simulink model "LATC_Test_Calc"  (R2021b)
settings: Solver=FixedStepDiscrete  StartTime=3849.7586  StopTime=3889.7825  FixedStep=0.01  RelTol=1e-3
values from neighbouring files (symbols this model uses):
  P_Global_CharSpd_ms : value not decoded    [PubParsGlobal.sldd]
  P_Global_SteeringAngleRatio : value not decoded    [PubParsGlobal.sldd]
  P_Global_WheelBase_m : value not decoded    [PubParsGlobal.sldd]
  P_LCS_CycleTime = 0.4 0.4 0.4 0.4 0.4 0.4 0.4 0.4 0.4 0.6 0.6 0.6 0.6 0.6 0.6 0.6 0.4 0.4 0.4 0.4 0.4 0.4 0.4 0.4 0.4 0.6 0.6 0.6 0.6 0.6 0.6 0.6 0.4 0.4 0.4 0.4 0.4 0.4 0.4 0.4 0.4 0.6 0.6 0.6 0.6 0.6 0.6 0.6 0.4 0.4 0.4 0.4 0.4 0.4 0.4 0.4 0.4 0.6 0.6 0.6 0.6 0.6 0.6 0.6 0.4 0.4 0.4 0.4 0.4 0.4 0.4 0.4 0.4 0.6 0.6 0.6 0.6 0.6 0.6 0.6 0.4 0.4 0.4 0.4 0.4 0.4 0.4 0.4 0.4 0.6 0.6 0.6 0.6 0.6 0.6 0.6 0.4 0.4 0.4 0.4    [LATC.sldd]
  P_LCS_ESS_AngleSlope_Limit = 2.9    [LATC.sldd]    (also in LCS_v05.sldd)
  P_LCS_LATC_CurOffsetVehicleSpdLimitValue_degs = 7.0    [LATC.sldd]
  P_LCS_LATC_ELKAngleSlope_ratio : value not decoded    [LATC.sldd]
  P_LCS_LATC_ELKMaxLatAcc_ms2 : value not decoded    [LATC.sldd]
  P_LCS_LATC_ESSAngleSlope_ratio : value not decoded    [LATC.sldd]
  P_LCS_LATC_ESSMaxLatAcc_ms2 : value not decoded    [LATC.sldd]
  P_LCS_LATC_LCAngleSlope_ratio : value not decoded    [LATC.sldd]
  P_LCS_LATC_LCCancleMaxLatAcc_ms2 : value not decoded    [LATC.sldd]
  P_LCS_LATC_LCEcoAngleSlope_ratio : value not decoded    [LATC.sldd]
  P_LCS_LATC_LCEcoMaxLatAcc_ms2 : value not decoded    [LATC.sldd]
  P_LCS_LATC_LCKAngleSlope_ratio : value not decoded    [LATC.sldd]
  P_LCS_LATC_LCKIEAngleSlope_ratio : value not decoded    [LATC.sldd]
  P_LCS_LATC_LCKIEMaxLatAcc_ms2 : value not decoded    [LATC.sldd]
  P_LCS_LATC_LCKMaxLatAcc_ms2 : value not decoded    [LATC.sldd]
  P_LCS_LATC_LCNormalAngleSlope_ratio : value not decoded    [LATC.sldd]
  P_LCS_LATC_LCNormalMaxLatAcc_ms2 : value not decoded    [LATC.sldd]
  P_LCS_LATC_LCSportAngleSlope_ratio : value not decoded    [LATC.sldd]
  P_LCS_LATC_LCSportMaxLatAcc_ms2 : value not decoded    [LATC.sldd]
  P_LCS_LATC_LKAAngleSlope_ratio : value not decoded    [LATC.sldd]
  P_LCS_LATC_LKAMaxLatAcc_ms2 : value not decoded    [LATC.sldd]
  P_LCS_LATC_MatrixQ1_st = 0.8 0.8 1.2 1.4 1.4 1.4 2.0 2.2 2.2 2.2 2.2 2.2 2.2 2.2 2.2 2.2 0.8 0.8 1.2 1.4 1.4 1.4 2.0 2.2 2.2 2.2 2.2 2.2 2.2 2.2 2.2 2.2 0.8 0.8 1.2 1.4 1.4 1.4 2.0 2.2 2.2 2.2 2.2 2.2 2.2 2.2 2.2 2.2 0.8 0.8 1.2 1.4 1.4 1.4 2.0 2.2 2.2 2.2 2.2 2.2 2.2 2.2 2.2 2.2 0.8 0.8 1.2 1.4 1.4 1.4 2.0 2.2 2.2 2.2 2.2 2.2 2.2 2.2 2.2 2.2 0.8 0.8 1.2 1.4 1.4 1.4 2.0 2.2 2.2 2.2 2.2 2.2 2.2 2.2 2.2 2.2 0.8 0.8 1.2 1.4    [LATC.sldd]
  P_LCS_LATC_MatrixQ3_st = 20.0 20.0 20.0 20.0 20.0 15.0 15.0 15.0 15.0 15.0 15.0 15.0 15.0 13.0 13.0 13.0 20.0 20.0 20.0 20.0 20.0 15.0 15.0 15.0 15.0 15.0 15.0 15.0 15.0 13.0 13.0 13.0 20.0 20.0 20.0 20.0 20.0 15.0 15.0 15.0 15.0 15.0 15.0 15.0 15.0 13.0 13.0 13.0 20.0 20.0 20.0 20.0 20.0 15.0 15.0 15.0 15.0 15.0 15.0 15.0 15.0 13.0 13.0 13.0 20.0 20.0 20.0 20.0 20.0 15.0 15.0 15.0 15.0 15.0 15.0 15.0 15.0 13.0 13.0 13.0    [LATC.sldd]
  P_LCS_LATC_MatrixR_st = 10.0 10.0 10.0 10.0 10.0 10.0 10.0 15.0 15.0 15.0 15.0 15.0 15.0 15.0 15.0 15.0 10.0 10.0 10.0 10.0 10.0 10.0 10.0 15.0 15.0 15.0 15.0 15.0 15.0 15.0 15.0 15.0 10.0 10.0 10.0 10.0 10.0 10.0 10.0 15.0 15.0 15.0 15.0 15.0 15.0 15.0 15.0 15.0 10.0 10.0 10.0 10.0 10.0 10.0 10.0 15.0 15.0 15.0 15.0 15.0 15.0 15.0 15.0 15.0 10.0 10.0 10.0 10.0 10.0 10.0 10.0 15.0 15.0 15.0 15.0 15.0 15.0 15.0 15.0 15.0    [LATC.sldd]
  P_LCS_LATC_StateActivAngleSlopeLimit_ratio : value not decoded    [LATC.sldd]
  P_LCS_LATC_StateActiveFlg_TabX_st : value not decoded    [LATC.sldd]
  P_LCS_LATC_StateActiveHoldTime_TabY_st : value not decoded    [LATC.sldd]
  P_LCS_LATC_StateHoldTime_st = 250.0    [LATC.sldd]
  P_LCS_LATC_TarAngleFliterWindowSize = 5.0    [LATC.sldd]
  P_LCS_LineVaildSW = 0.0    [LATC.sldd]
  P_LCS_Lookahead_Distance : value not decoded    [LATC.sldd]
  P_LCS_VehicleSpd_TabX_Kph : value not decoded    [LATC.sldd]
libraries: simulink x4
(part 2 of 4)

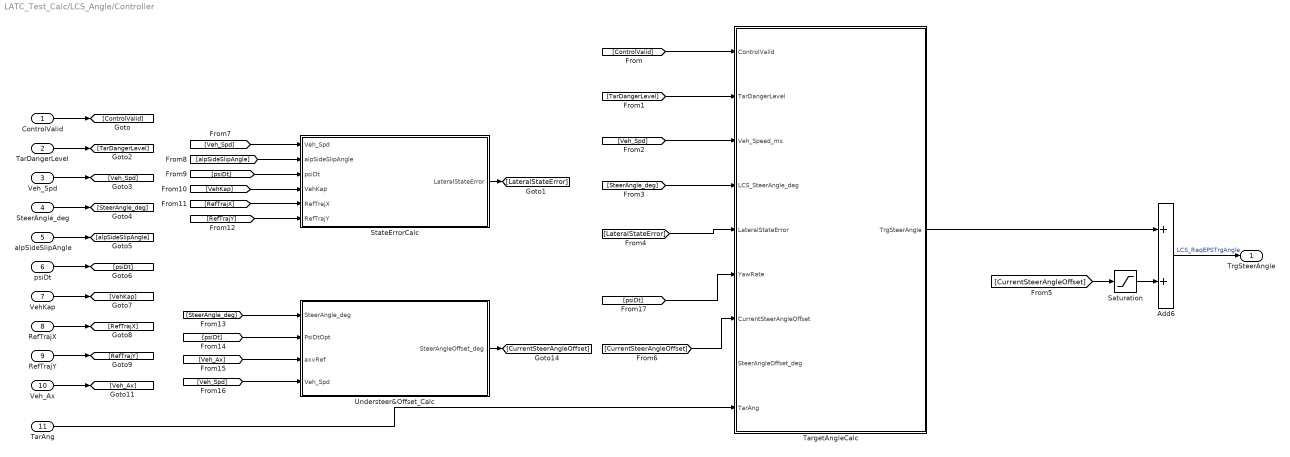
== system LATC_Test_Calc/LCS_Angle/Controller ==
  ControlValid : Inport
  TarDangerLevel : Inport  Port=2
  Veh_Spd : Inport  Port=3
  SteerAngle_deg : Inport  Port=4
  alpSideSlipAngle : Inport  Port=5
  psiDt : Inport  Port=6
  VehKap : Inport  Port=7
  RefTrajX : Inport  Port=8
  RefTrajY : Inport  Port=9
  Veh_Ax : Inport  Port=10
  TarAng : Inport  Port=11
  Add6 : Sum  AccumDataTypeStr=single
  Saturation : Saturate  UpperLimit=10  LowerLimit=-10
  StateErrorCalc : Subsystem
  TargetAngleCalc : Subsystem
  Understeer&Offset_Calc : Subsystem
  TrgSteerAngle : Outport
  wires:
  Understeer&Offset_Calc/1(SteerAngleOffset_deg) -> [CurrentSteerAngleOffset]
  StateErrorCalc/1(LateralStateError) -> [LateralStateError]
  ControlValid/1 -> [ControlValid]
  TarDangerLevel/1 -> [TarDangerLevel]
  Veh_Spd/1 -> [Veh_Spd]
  SteerAngle_deg/1 -> [SteerAngle_deg]
  alpSideSlipAngle/1 -> [alpSideSlipAngle]
  psiDt/1 -> [psiDt]
  VehKap/1 -> [VehKap]
  RefTrajX/1 -> [RefTrajX]
  RefTrajY/1 -> [RefTrajY]
  [ControlValid] -> TargetAngleCalc/1(ControlValid)
  [TarDangerLevel] -> TargetAngleCalc/2(TarDangerLevel)
  [Veh_Spd] -> TargetAngleCalc/3(Veh_Speed_ms)
  [SteerAngle_deg] -> TargetAngleCalc/4(LCS_SteerAngle_deg)
  [LateralStateError] -> TargetAngleCalc/5(LateralStateError)
  [psiDt] -> TargetAngleCalc/6(YawRate)
  [CurrentSteerAngleOffset] -> TargetAngleCalc/7(CurrentSteerAngleOffset)
  [Veh_Spd] -> StateErrorCalc/1(Veh_Spd)
  [alpSideSlipAngle] -> StateErrorCalc/2(alpSideSlipAngle)
  [psiDt] -> StateErrorCalc/3(psiDt)
  [VehKap] -> StateErrorCalc/4(VehKap)
  [RefTrajX] -> StateErrorCalc/5(RefTrajX)
  [RefTrajY] -> StateErrorCalc/6(RefTrajY)
  [SteerAngle_deg] -> Understeer&Offset_Calc/1(SteerAngle_deg)
  [psiDt] -> Understeer&Offset_Calc/2(PsiDtOpt)
  Veh_Ax/1 -> [Veh_Ax]
  [Veh_Ax] -> Understeer&Offset_Calc/3(axvRef)
  [Veh_Spd] -> Understeer&Offset_Calc/4(Veh_Spd)
  [CurrentSteerAngleOffset] -> Saturation/1
  Saturation/1 -> Add6/2
  TargetAngleCalc/1(TrgSteerAngle) -> Add6/1
  Add6/1 -> TrgSteerAngle/1  "LCS_ReqEPSTrgAngle"
  TarAng/1 -> TargetAngleCalc/9(TarAng)

== system LATC_Test_Calc/LCS_Angle/LaneWidthFac ==
  LaneWidth : Inport
  Constant4 : Constant  Value=3.6  OutDataTypeStr=single
  Constant6 : Constant  Value=3  OutDataTypeStr=single
  Constant7 : Constant  Value=4  OutDataTypeStr=single
  Divide1 : Product  Inputs=*/
  MinMax : MinMax  Function=max  Inputs=2
  MinMax1 : MinMax  Inputs=2
  LaneWidthFac : Outport
  wires:
  LaneWidth/1 -> MinMax/1
  Constant7/1 -> MinMax1/2
  MinMax/1 -> MinMax1/1
  Constant6/1 -> MinMax/2
  Constant4/1 -> Divide1/2
  MinMax1/1 -> Divide1/1
  Divide1/1 -> LaneWidthFac/1

== system LATC_Test_Calc/LCS_Angle/Subsystem ==
  canSteerWheelSpd : Inport
  canSteerWheelSpdSign : Inport  Port=2
  Bias2 : Bias  Bias=-0.5
  Gain2 : Gain  Gain=-2
  Product4 : Product
  LCS_IN_SteerAngleSpd_degs : Outport
  wires:
  Gain2/1 -> Product4/2
  Product4/1 -> LCS_IN_SteerAngleSpd_degs/1
  canSteerWheelSpdSign/1 -> Bias2/1
  Bias2/1 -> Gain2/1
  canSteerWheelSpd/1 -> Product4/1

== system LATC_Test_Calc/LCS_Angle/Subsystem1 ==
  Speed_ms : Inport
  Constant8 : Constant  Value=1.3  OutDataTypeStr=single
  Gain3 : Gain  Gain=3.6
  Gain4 : Gain  Gain=1.03
  Sum : Sum
  LCS_DisplaySpd_kph : Outport
  wires:
  Constant8/1 -> Sum/2
  Speed_ms/1 -> Gain3/1
  Gain3/1 -> Gain4/1
  Sum/1 -> LCS_DisplaySpd_kph/1
  Gain4/1 -> Sum/1

== system LATC_Test_Calc/LCS_Angle/Subsystem3 ==
  canSteerWheelAngle : Inport
  canSteerWheelAngleSign : Inport  Port=2
  Bias1 : Bias  Bias=-0.5
  Gain5 : Gain  Gain=-2
  Product5 : Product
  LCS_IN_CurSteerAngle_deg : Outport
  wires:
  Bias1/1 -> Gain5/1
  canSteerWheelAngle/1 -> Product5/1
  Gain5/1 -> Product5/2
  canSteerWheelAngleSign/1 -> Bias1/1
  Product5/1 -> LCS_IN_CurSteerAngle_deg/1  "LCS_IN_CurSteerAngle_deg"

== system LATC_Test_Calc/LCS_Angle/Subsystem5 ==
  raw : Inport
  Slope : Inport  Port=2
  Add : Sum
  Add1 : Sum  Inputs=+-
  Max : MinMax  Inputs=2
  Min : MinMax  Function=max  Inputs=2
  Unit Delay : UnitDelay  InitialCondition=single(0)  SampleTime=-1  HasFrameUpgradeWarning=on
  out : Outport
  wires:
  raw/1 -> Max/2
  Add1/1 -> Min/2
  Add/1 -> Max/1
  Max/1 -> Min/1
  Min/1 -> Unit Delay/1, out/1
  Unit Delay/1 -> Add/1, Add1/1
  Slope/1 -> Add/2, Add1/2

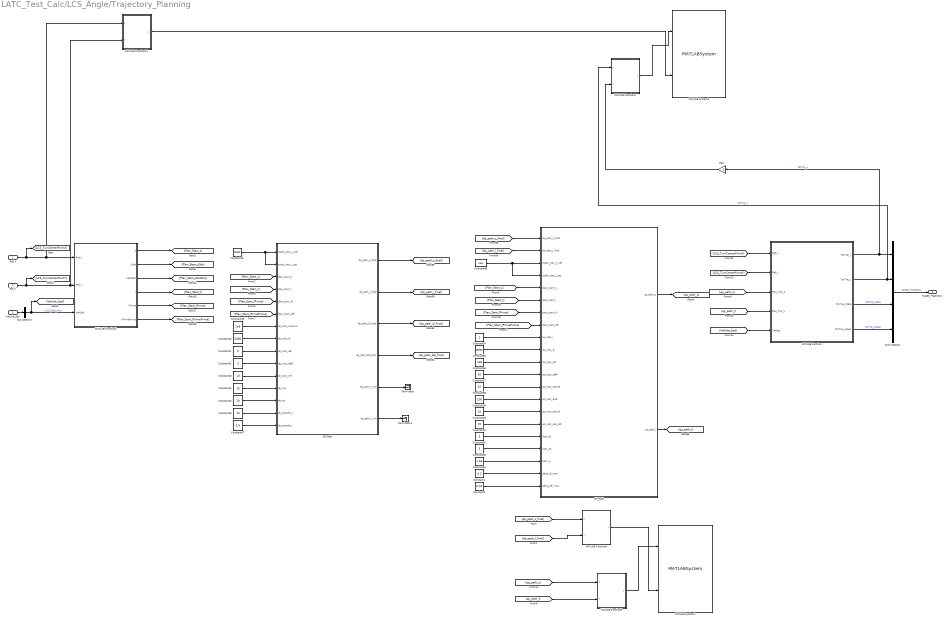
== system LATC_Test_Calc/LCS_Angle/Trajectory_Planning ==
  Ref_X : Inport
  Ref_Y : Inport  Port=2
  Vehicle_Spd : Inport  Port=3
  Bus Creator1 : BusCreator  Inputs=4
  Bus Selector : BusSelector  OutputSignals=LCS_Spd_ms
  Constant1 : Constant  Value=0.2  OutDataTypeStr=single
  Constant2 : Constant  Value=0.01  OutDataTypeStr=single
  Constant39 : Constant  Value=1e9  OutDataTypeStr=single
  Constant40 : Constant  Value=2000  OutDataTypeStr=single
  Constant41 : Constant  Value=2  OutDataTypeStr=single
  Constant42 : Constant  Value=3  OutDataTypeStr=single
  Constant43 : Constant  Value=10  OutDataTypeStr=single
  Constant{44,58,60..61} (4 alike) : Constant  Value=15  OutDataTypeStr=single
  Constant45 : Constant  Value=10  OutDataTypeStr=single
  Constant46 : Constant  Value=12  OutDataTypeStr=single
  Constant47 : Constant  Value=0.5  OutDataTypeStr=single
  Constant49 : Constant  Value=NaN  OutDataTypeStr=single
  Constant54 : Constant  OutDataTypeStr=single
  Constant55 : Constant  Value=25000  OutDataTypeStr=single
  Constant56 : Constant  Value=100  OutDataTypeStr=single
  Constant57 : Constant  Value=20  OutDataTypeStr=single
  Constant59 : Constant  Value=100  OutDataTypeStr=single
  Constant62 : Constant  Value=3  OutDataTypeStr=single
  Constant63 : Constant  Value=3  OutDataTypeStr=single
  Constant64 : Constant  Value=1.63  OutDataTypeStr=single
  Constant68 : Constant  Value=nan  OutDataTypeStr=single
  DP_Path : Subsystem
  Gain : Gain  Gain=-1
  MATLAB Function : MATLAB Function  TreatAsAtomicUnit=on
  MATLAB Function1 : MATLAB Function  TreatAsAtomicUnit=on
  MATLAB Function14 : MATLAB Function  TreatAsAtomicUnit=on
  MATLAB Function2 : MATLAB Function  TreatAsAtomicUnit=on
  MATLAB Function3 : MATLAB Function  TreatAsAtomicUnit=on
  MATLAB Function4 : MATLAB Function  TreatAsAtomicUnit=on
  MATLAB System1 : MATLABSystem  System=BirdsEyeView17a  XLim=[ 0, 120 ]  YLim=[ -30, 30 ]  HasActors=off  ActorsColor=off  HasVision=on  HasRadar=on  HasRoads=off  HasLaneMarkings=off  Camera_Fov=52  Camera_Range=100  Camera_Yaw=0  Camera_Pos=[ 0, 0 ]  Radar_Fov=52  Radar_Range=100  Radar_Yaw=0  Radar_Pos=[ 0, 0 ]  MarkerSize=4  LabelFontSize=4  LabelOffset=[ 1.5, 1.5 ]  aspectratio=off
      mask Type: BirdsEyeView17a
      mask Display:
      | disp(['Bird''s-Eye' char(10) 'View']);
      | port_label('input',1,'Vision');
      | port_label('input',2,'Radar');
  MATLAB System3 : MATLABSystem  System=BirdsEyeView17a  XLim=[ 0, 120 ]  YLim=[ -30, 30 ]  HasActors=off  ActorsColor=off  HasVision=on  HasRadar=on  HasRoads=off  HasLaneMarkings=off  Camera_Fov=52  Camera_Range=100  Camera_Yaw=0  Camera_Pos=[ 0, 0 ]  Radar_Fov=52  Radar_Range=100  Radar_Yaw=0  Radar_Pos=[ 0, 0 ]  MarkerSize=4  LabelFontSize=4  LabelOffset=[ 1.5, 1.5 ]  aspectratio=off
      mask Type: BirdsEyeView17a
      mask Display:
      | disp(['Bird''s-Eye' char(10) 'View']);
      | port_label('input',1,'Vision');
      | port_label('input',2,'Radar');
  QP_Path : Subsystem
  Terminator : Terminator
  Terminator1 : Terminator
  Target_Trajectory : Outport
  wires:
  Constant55/1 -> QP_Path/10(qp_cost_dl)
  MATLAB Function2/6(lPrimePrime) -> [Plan_Start_lPrimePrime]
  MATLAB Function2/1(s) -> [Plan_Start_s]
  Constant41/1 -> DP_Path/9(dp_cost_ddl)
  Constant56/1 -> QP_Path/11(qp_cost_ddl)
  QP_Path/2(qp_path_l) -> [qp_path_l]
  [Plan_Start_lPrime] -> DP_Path/5(plan_start_dl)
  Constant62/1 -> QP_Path/17(host_d1)
  Constant61/1 -> QP_Path/16(qp_cost_end_ddl)
  [Plan_Start_lPrimePrime] -> DP_Path/6(plan_start_ddl)
  Constant54/1 -> QP_Path/9(qp_cost_l)
  Constant42/1 -> DP_Path/10(dp_cost_dddl)
  Vehicle_Spd/1 -> Bus Selector/1
  [Plan_Start_lPrimePrime] -> QP_Path/8(plan_start_ddl)
  Constant59/1 -> QP_Path/14(qp_cost_endl)
  Constant68/1 -> QP_Path/4(static_obs_l_set), QP_Path/3(static_obs_s_set)
  Constant44/1 -> DP_Path/12(dp_row)
  [Plan_Start_l] -> DP_Path/4(plan_start_l)
  MATLAB Function2/5(lPrime) -> [Plan_Start_lPrime]
  [Plan_Start_s] -> DP_Path/3(plan_start_s)
  DP_Path/1(dp_path_s_final) -> [dp_path_s_final]
  [dp_path_s_final] -> QP_Path/1(dp_path_s_final)
  Constant64/1 -> QP_Path/19(host_w)
  MATLAB Function2/3(sDotDot) -> [Plan_Start_sDotDot]
  Constant46/1 -> DP_Path/14(dp_sample_s)
  [Vehicle_Spd] -> MATLAB Function/5(VehSpd)
  Constant63/1 -> QP_Path/18(host_d2)
  DP_Path/3(dp_path_dl_final) -> [dp_path_dl_final]
  DP_Path/2(dp_path_l_final) -> [dp_path_l_final]
  Constant40/1 -> DP_Path/8(dp_cost_dl)
  Constant57/1 -> QP_Path/12(qp_cost_dddl)
  Constant47/1 -> DP_Path/15(dp_sample_l)
  MATLAB Function2/4(l) -> [Plan_Start_l]
  MATLAB Function2/2(sDot) -> [Plan_Start_sDot]
  Constant39/1 -> DP_Path/7(dp_cost_collision)
  Constant43/1 -> DP_Path/11(dp_cost_ref)
  [Plan_Start_lPrime] -> QP_Path/7(plan_start_dl)
  MATLAB Function/1(TarTraj_x) -> Gain/1, Bus Creator1/1  "TarTraj_x"
  DP_Path/4(dp_path_ddl_final) -> [dp_path_ddl_final]
  Constant60/1 -> QP_Path/15(qp_cost_end_dl)
  [LCS_TurnCenterPointY] -> MATLAB Function/2(Ref_Y)
  Bus Selector/1 -> [Vehicle_Spd], MATLAB Function2/3(VehSpd)  "<LCS_Spd_ms>"
  [Plan_Start_l] -> QP_Path/6(plan_start_l)
  [qp_path_s] -> MATLAB Function/3(Plan_Traj_S)
  DP_Path/6(dp_path_l_init) -> Terminator1/1
  Constant49/1 -> DP_Path/2(static_obs_l_set), DP_Path/1(static_obs_s_set)
  Constant58/1 -> QP_Path/13(qp_cost_centre)
  [dp_path_l_final] -> QP_Path/2(dp_path_l_final)
  DP_Path/5(dp_path_s_init) -> Terminator/1
  Constant45/1 -> DP_Path/13(dp_col)
  [qp_path_l] -> MATLAB Function/4(Plan_Traj_L)
  Bus Creator1/1 -> Target_Trajectory/1  "Target_Trajectory"
  [LCS_TurnCenterPointX] -> MATLAB Function/1(Ref_X)
  MATLAB Function/4(TarTraj_kappa) -> Bus Creator1/4  "TarTraj_kappa"
  MATLAB Function/2(TarTraj_y) -> MATLAB Function1/1(X), Bus Creator1/2  "TarTraj_y"
  MATLAB Function/3(TarTraj_theta) -> Bus Creator1/3  "TarTraj_theta"
  Ref_X/1 -> [LCS_TurnCenterPointX], MATLAB Function14/1(X), MATLAB Function2/1(Ref_X)
  MATLAB Function1/1(y) -> MATLAB System3/1
  Ref_Y/1 -> [LCS_TurnCenterPointY], MATLAB Function14/2(Y), MATLAB Function2/2(Ref_Y)
  MATLAB Function14/1(y) -> MATLAB System3/2
  Gain/1 -> MATLAB Function1/2(Y)
  [dp_path_l_final] -> MATLAB Function4/2(Y)
  MATLAB Function3/1(y) -> MATLAB System1/1
  [dp_path_s_final] -> MATLAB Function4/1(X)
  MATLAB Function4/1(y) -> MATLAB System1/2
  Constant1/1 -> QP_Path/20(delta_dl_max)
  Constant2/1 -> QP_Path/21(delta_ddl_max)
  QP_Path/1(qp_path_s) -> [qp_path_s]
  [Plan_Start_s] -> QP_Path/5(plan_start_s)
  [qp_path_s] -> MATLAB Function3/1(X)
  [qp_path_l] -> MATLAB Function3/2(Y)

== system LATC_Test_Calc/LCS_Angle/Trajectory_Points ==
  A0 : Inport
  A1 : Inport  Port=2
  A2 : Inport  Port=3
  A3 : Inport  Port=4
  LineVaild : Inport  Port=5
  MATLAB Function1 : MATLAB Function  TreatAsAtomicUnit=on
  RoadCreate1 : Subsystem
  LCS_TurnCenterPointX : Outport
  LCS_TurnCenterPointY : Outport  Port=2
  Control_Valid : Outport  Port=3
  wires:
  A1/1 -> RoadCreate1/2(A1)
  MATLAB Function1/2(CenterLinePoint2_Y) -> LCS_TurnCenterPointY/1  "LCS_TurnCenterPointY"
  A0/1 -> RoadCreate1/1(A0)
  MATLAB Function1/1(CenterLinePoint2_X) -> LCS_TurnCenterPointX/1  "LCS_TurnCenterPointX"
  A2/1 -> RoadCreate1/3(A2)
  LineVaild/1 -> RoadCreate1/5(LineVaild)
  RoadCreate1/3(Control_Valid) -> Control_Valid/1
  A3/1 -> RoadCreate1/4(A3)
  RoadCreate1/1(CenterLinePointX) -> MATLAB Function1/1(CenterLinePointX)
  RoadCreate1/2(CenterLinePointY) -> MATLAB Function1/2(CenterLinePointY)

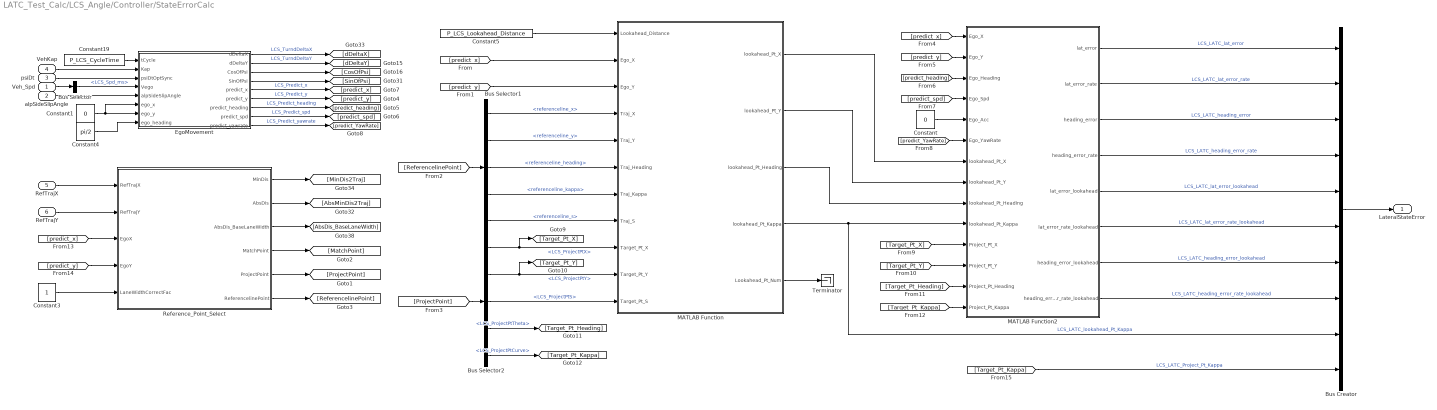
== system LATC_Test_Calc/LCS_Angle/Controller/StateErrorCalc ==
  Veh_Spd : Inport
  alpSideSlipAngle : Inport  Port=2
  psiDt : Inport  Port=3
  VehKap : Inport  Port=4
  RefTrajX : Inport  Port=5
  RefTrajY : Inport  Port=6
  Bus Creator : BusCreator  Inputs=10
  Bus Selector : BusSelector  OutputSignals=LCS_Spd_ms
  Bus Selector1 : BusSelector  OutputSignals=referenceline_x,referenceline_y,referenceline_heading,referenceline_kappa,referenceline_s
  Bus Selector2 : BusSelector  OutputSignals=LCS_ProjectPtX,LCS_ProjectPtY,LCS_ProjectPtS,LCS_ProjectPtTheta,LCS_ProjectPtCurve
  Constant : Constant  Value=0  OutDataTypeStr=single
  Constant1 : Constant  Value=0  OutDataTypeStr=single
  Constant19 : Constant  Value=P_LCS_CycleTime  OutDataTypeStr=single
  Constant3 : Constant  OutDataTypeStr=single
  Constant4 : Constant  Value=pi/2  OutDataTypeStr=single
  Constant5 : Constant  Value=P_LCS_Lookahead_Distance  OutDataTypeStr=single
  EgoMovement : MATLAB Function  TreatAsAtomicUnit=on
  MATLAB Function : MATLAB Function  TreatAsAtomicUnit=on
  MATLAB Function2 : MATLAB Function  TreatAsAtomicUnit=on
  Reference_Point_Select : Subsystem
  Terminator : Terminator
  LateralStateError : Outport
  wires:
  Constant19/1 -> EgoMovement/1(tCycle)
  Bus Selector/1 -> EgoMovement/4(Vego)  "<LCS_Spd_ms>"
  EgoMovement/1(dDeltaX) -> [dDeltaX]  "LCS_TurndDeltaX"
  EgoMovement/4(SinOfPsi) -> [SinOfPsi]
  VehKap/1 -> EgoMovement/2(Kap)
  EgoMovement/3(CosOfPsi) -> [CosOfPsi]
  Veh_Spd/1 -> Bus Selector/1
  alpSideSlipAngle/1 -> EgoMovement/5(alpSideSlipAngle)
  psiDt/1 -> EgoMovement/3(psiDtOptSync)
  EgoMovement/2(dDeltaY) -> [dDeltaY]  "LCS_TurndDeltaY"
  Reference_Point_Select/3(AbsDis_BaseLaneWidth) -> [AbsDis_BaseLaneWidth]
  Reference_Point_Select/2(AbsDis) -> [AbsMinDis2Traj]
  Reference_Point_Select/1(MinDis) -> [MinDis2Traj]
  RefTrajX/1 -> Reference_Point_Select/1(RefTrajX)
  Constant3/1 -> Reference_Point_Select/5(LaneWidthCorrectFac)
  RefTrajY/1 -> Reference_Point_Select/2(RefTrajY)
  Reference_Point_Select/4(MatchPoint) -> [MatchPoint]
  Reference_Point_Select/5(ProjectPoint) -> [ProjectPoint]
  Reference_Point_Select/6(ReferencelinePoint) -> [ReferencelinePoint]
  EgoMovement/5(predict_x) -> [predict_x]  "LCS_Predict_x"
  EgoMovement/6(predict_y) -> [predict_y]  "LCS_Predict_y"
  EgoMovement/7(predict_heading) -> [predict_heading]  "LCS_Predict_heading"
  EgoMovement/8(predict_spd) -> [predict_spd]  "LCS_Predict_spd"
  EgoMovement/9(predict_yawrate) -> [predict_YawRate]  "LCS_Predict_yawrate"
  [predict_x] -> MATLAB Function/2(Ego_X)
  [predict_y] -> MATLAB Function/3(Ego_Y)
  [ReferencelinePoint] -> Bus Selector1/1
  Bus Selector1/1 -> MATLAB Function/4(Traj_X)  "<referenceline_x>"
  Bus Selector1/2 -> MATLAB Function/5(Traj_Y)  "<referenceline_y>"
  Bus Selector1/3 -> MATLAB Function/6(Traj_Heading)  "<referenceline_heading>"
  Bus Selector1/4 -> MATLAB Function/7(Traj_Kappa)  "<referenceline_kappa>"
  Bus Selector1/5 -> MATLAB Function/8(Traj_S)  "<referenceline_s>"
  [ProjectPoint] -> Bus Selector2/1
  Bus Selector2/2 -> [Target_Pt_Y], MATLAB Function/10(Target_Pt_Y)  "<LCS_ProjectPtY>"
  Bus Selector2/1 -> [Target_Pt_X], MATLAB Function/9(Target_Pt_X)  "<LCS_ProjectPtX>"
  Bus Selector2/3 -> MATLAB Function/11(Target_Pt_S)  "<LCS_ProjectPtS>"
  [predict_x] -> MATLAB Function2/1(Ego_X)
  [predict_y] -> MATLAB Function2/2(Ego_Y)
  [predict_heading] -> MATLAB Function2/3(Ego_Heading)
  [predict_spd] -> MATLAB Function2/4(Ego_Spd)
  [predict_YawRate] -> MATLAB Function2/6(Ego_YawRate)
  Constant/1 -> MATLAB Function2/5(Ego_Acc)
  Bus Selector2/4 -> [Target_Pt_Heading]  "<LCS_ProjectPtTheta>"
  Bus Selector2/5 -> [Target_Pt_Kappa]  "<LCS_ProjectPtCurve>"
  [Target_Pt_X] -> MATLAB Function2/11(Project_Pt_X)
  [Target_Pt_Y] -> MATLAB Function2/12(Project_Pt_Y)
  [Target_Pt_Heading] -> MATLAB Function2/13(Project_Pt_Heading)
  [Target_Pt_Kappa] -> MATLAB Function2/14(Project_Pt_Kappa)
  Constant1/1 -> EgoMovement/7(ego_y), EgoMovement/6(ego_x)
  MATLAB Function2/4(heading_error_rate) -> Bus Creator/4  "LCS_LATC_heading_error_rate"
  MATLAB Function2/2(lat_error_rate) -> Bus Creator/2  "LCS_LATC_lat_error_rate"
  MATLAB Function2/3(heading_error) -> Bus Creator/3  "LCS_LATC_heading_error"
  MATLAB Function2/1(lat_error) -> Bus Creator/1  "LCS_LATC_lat_error"
  Bus Creator/1 -> LateralStateError/1
  Constant4/1 -> EgoMovement/8(ego_heading)
  MATLAB Function/4(lookahead_Pt_Kappa) -> Bus Creator/9, MATLAB Function2/10(lookahead_Pt_Kappa)  "LCS_LATC_lookahead_Pt_Kappa"
  Constant5/1 -> MATLAB Function/1(Lookahead_Distance)
  [predict_x] -> Reference_Point_Select/3(EgoX)
  [predict_y] -> Reference_Point_Select/4(EgoY)
  MATLAB Function/5(Lookahead_Pt_Num) -> Terminator/1
  MATLAB Function/2(lookahead_Pt_Y) -> MATLAB Function2/8(lookahead_Pt_Y)
  MATLAB Function/1(lookahead_Pt_X) -> MATLAB Function2/7(lookahead_Pt_X)
  MATLAB Function/3(lookahead_Pt_Heading) -> MATLAB Function2/9(lookahead_Pt_Heading)
  MATLAB Function2/5(lat_error_lookahead) -> Bus Creator/5  "LCS_LATC_lat_error_lookahead"
  MATLAB Function2/6(lat_error_rate_lookahead) -> Bus Creator/6  "LCS_LATC_lat_error_rate_lookahead"
  MATLAB Function2/7(heading_error_lookahead) -> Bus Creator/7  "LCS_LATC_heading_error_lookahead"
  MATLAB Function2/8(heading_error_rate_lookahead) -> Bus Creator/8  "LCS_LATC_heading_error_rate_lookahead"
  [Target_Pt_Kappa] -> Bus Creator/10  "LCS_LATC_Project_Pt_Kappa"

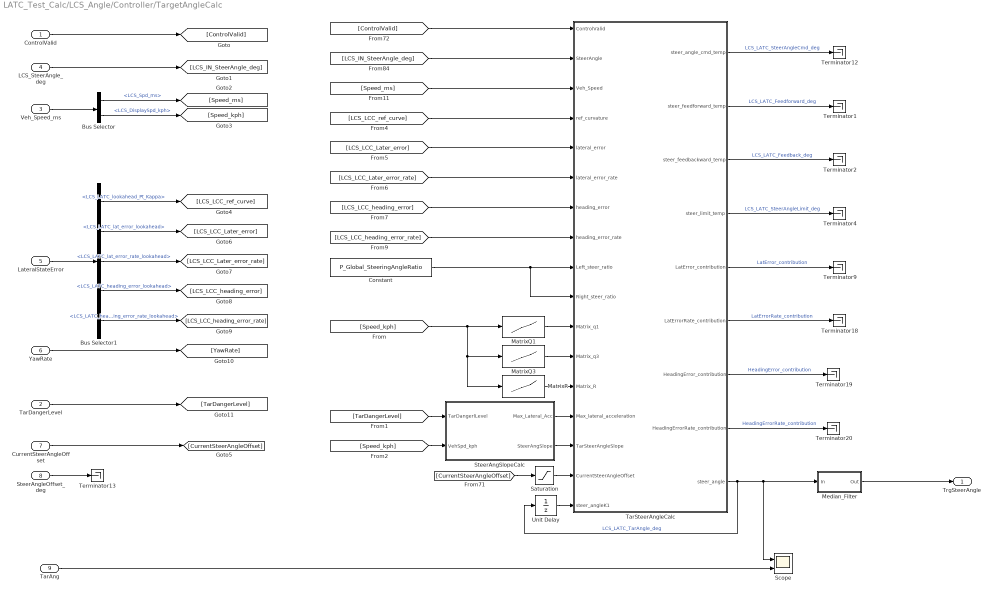
== system LATC_Test_Calc/LCS_Angle/Controller/TargetAngleCalc ==
  ControlValid : Inport
  TarDangerLevel : Inport  Port=2
  Veh_Speed_ms : Inport  Port=3
  LCS_SteerAngle_deg : Inport  Port=4
  LateralStateError : Inport  Port=5
  YawRate : Inport  Port=6
  CurrentSteerAngleOffset : Inport  Port=7
  SteerAngleOffset_deg : Inport  Port=8
  TarAng : Inport  Port=9
  Bus Selector : BusSelector  OutputSignals=LCS_Spd_ms,LCS_DisplaySpd_kph
  Bus Selector1 : BusSelector  OutputSignals=LCS_LATC_lookahead_Pt_Kappa,LCS_LATC_lat_error_lookahead,LCS_LATC_lat_error_rate_lookahead,LCS_LATC_heading_error_lookahead,LCS_LATC_heading_error_rate_lookahead
  Constant : Constant  Value=P_Global_SteeringAngleRatio  OutDataTypeStr=single
  MatrixQ1 : Lookup_n-D  NumberOfTableDimensions=1  BreakpointsForDimension1=P_LCS_VehicleSpd_TabX_Kph  Table=P_LCS_LATC_MatrixQ1_st  ExtrapMethod=Clip  UseLastTableValue=on  InternalRulePriority=Speed  RndMeth=Simplest  InputSameDT=on
  MatrixQ3 : Lookup_n-D  NumberOfTableDimensions=1  BreakpointsForDimension1=P_LCS_VehicleSpd_TabX_Kph  Table=P_LCS_LATC_MatrixQ3_st  ExtrapMethod=Clip  UseLastTableValue=on  InternalRulePriority=Speed  RndMeth=Simplest  InputSameDT=on
  MatrixR : Lookup_n-D  NumberOfTableDimensions=1  BreakpointsForDimension1=P_LCS_VehicleSpd_TabX_Kph  Table=P_LCS_LATC_MatrixR_st  ExtrapMethod=Clip  UseLastTableValue=on  InternalRulePriority=Speed  RndMeth=Simplest  InputSameDT=on
  Median_Filter : Subsystem
  Saturation : Saturate  UpperLimit=8  LowerLimit=-8  OutDataTypeStr=single
  Scope : Scope  NumInputPorts=2
  SteerAngSlopeCalc : Subsystem
  TarSteerAngleCalc : MATLAB Function  TreatAsAtomicUnit=on
  Terminator{1..2,4,9,12..13,18..20} (9 alike) : Terminator
  Unit Delay : UnitDelay  SampleTime=-1  HasFrameUpgradeWarning=on
  TrgSteerAngle : Outport  OutDataTypeStr=single
  wires:
  [CurrentSteerAngleOffset] -> Saturation/1
  TarSteerAngleCalc/6(LatErrorRate_contribution) -> Terminator18/1  "LatErrorRate_contribution"
  SteerAngSlopeCalc/2(SteerAngSlope) -> TarSteerAngleCalc/15(TarSteerAngleSlope)
  TarSteerAngleCalc/8(HeadingErrorRate_contribution) -> Terminator20/1  "HeadingErrorRate_contribution"
  TarSteerAngleCalc/5(LatError_contribution) -> Terminator9/1  "LatError_contribution"
  TarSteerAngleCalc/9(steer_angle) -> Scope/1, Median_Filter/1(In), Unit Delay/1  "LCS_LATC_TarAngle_deg"
  TarSteerAngleCalc/4(steer_limit_temp) -> Terminator4/1  "LCS_LATC_SteerAngleLimit_deg"
  TarSteerAngleCalc/7(HeadingError_contribution) -> Terminator19/1  "HeadingError_contribution"
  [LCS_LCC_Later_error] -> TarSteerAngleCalc/5(lateral_error)
  Saturation/1 -> TarSteerAngleCalc/16(CurrentSteerAngleOffset)
  TarSteerAngleCalc/3(steer_feedbackward_temp) -> Terminator2/1  "LCS_LATC_Feedback_deg"
  MatrixQ3/1 -> TarSteerAngleCalc/12(Matrix_q3)
  TarSteerAngleCalc/2(steer_feedforward_temp) -> Terminator1/1  "LCS_LATC_Feedforward_deg"
  [Speed_kph] -> SteerAngSlopeCalc/2(VehSpd_kph)
  [ControlValid] -> TarSteerAngleCalc/1(ControlValid)
  MatrixR/1 -> TarSteerAngleCalc/13(Matrix_R)
  [LCS_LCC_heading_error] -> TarSteerAngleCalc/7(heading_error)
  [TarDangerLevel] -> SteerAngSlopeCalc/1(TarDangerlLevel)
  [LCS_LCC_Later_error_rate] -> TarSteerAngleCalc/6(lateral_error_rate)
  Constant/1 -> TarSteerAngleCalc/9(Left_steer_ratio), TarSteerAngleCalc/10(Right_steer_ratio)
  TarSteerAngleCalc/1(steer_angle_cmd_temp) -> Terminator12/1  "LCS_LATC_SteerAngleCmd_deg"
  [LCS_LCC_heading_error_rate] -> TarSteerAngleCalc/8(heading_error_rate)
  Median_Filter/1(Out) -> TrgSteerAngle/1
  MatrixQ1/1 -> TarSteerAngleCalc/11(Matrix_q1)
  [LCS_LCC_ref_curve] -> TarSteerAngleCalc/4(ref_curvature)
  [Speed_kph] -> MatrixR/1, MatrixQ3/1, MatrixQ1/1
  SteerAngSlopeCalc/1(Max_Lateral_Acc) -> TarSteerAngleCalc/14(Max_lateral_acceleration)
  [Speed_ms] -> TarSteerAngleCalc/3(Veh_Speed)
  [LCS_IN_SteerAngle_deg] -> TarSteerAngleCalc/2(SteerAngle)
  Unit Delay/1 -> TarSteerAngleCalc/17(steer_angleK1)
  LCS_SteerAngle_deg/1 -> [LCS_IN_SteerAngle_deg]
  SteerAngleOffset_deg/1 -> Terminator13/1
  ControlValid/1 -> [ControlValid]
  TarDangerLevel/1 -> [TarDangerLevel]
  YawRate/1 -> [YawRate]
  Veh_Speed_ms/1 -> Bus Selector/1
  Bus Selector/1 -> [Speed_ms]  "<LCS_Spd_ms>"
  Bus Selector/2 -> [Speed_kph]  "<LCS_DisplaySpd_kph>"
  LateralStateError/1 -> Bus Selector1/1
  Bus Selector1/2 -> [LCS_LCC_Later_error]  "<LCS_LATC_lat_error_lookahead>"
  Bus Selector1/3 -> [LCS_LCC_Later_error_rate]  "<LCS_LATC_lat_error_rate_lookahead>"
  Bus Selector1/4 -> [LCS_LCC_heading_error]  "<LCS_LATC_heading_error_lookahead>"
  Bus Selector1/5 -> [LCS_LCC_heading_error_rate]  "<LCS_LATC_heading_error_rate_lookahead>"
  CurrentSteerAngleOffset/1 -> [CurrentSteerAngleOffset]
  Bus Selector1/1 -> [LCS_LCC_ref_curve]  "<LCS_LATC_lookahead_Pt_Kappa>"
  TarAng/1 -> Scope/2

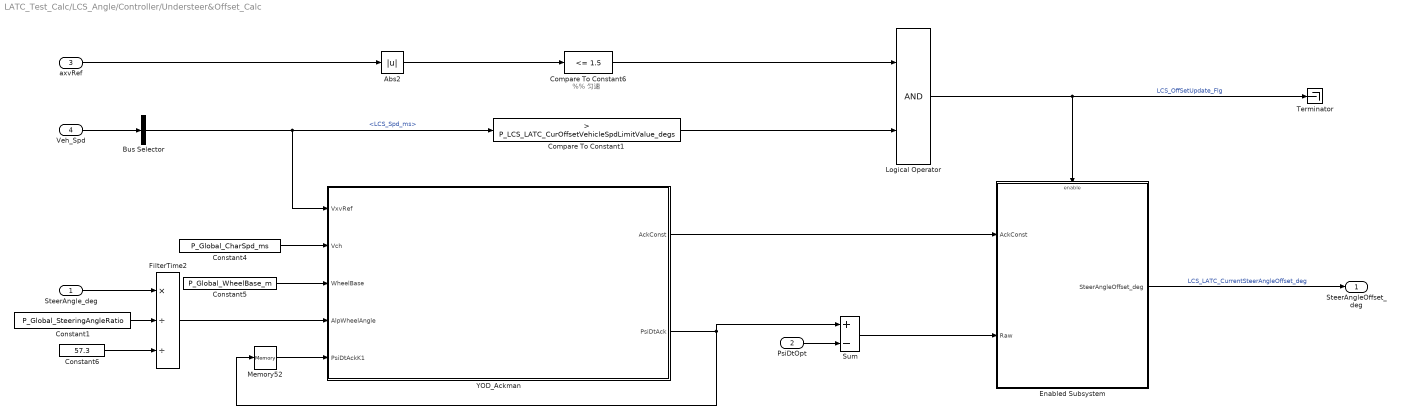
== system LATC_Test_Calc/LCS_Angle/Controller/Understeer&Offset_Calc ==
  note: %% 匀速
  SteerAngle_deg : Inport
  PsiDtOpt : Inport  Port=2
  axvRef : Inport  Port=3
  Veh_Spd : Inport  Port=4
  Abs2 : Abs
  Bus Selector : BusSelector  OutputSignals=LCS_Spd_ms
  Compare To Constant1 : simulink/Logic and Bit Operations/Compare To Constant  relop=>  const=P_LCS_LATC_CurOffsetVehicleSpdLimitValue_degs  OutDataTypeStr=boolean
  Compare To Constant6 : simulink/Logic and Bit Operations/Compare To Constant  relop=<=  const=1.5  OutDataTypeStr=boolean
  Constant1 : Constant  Value=P_Global_SteeringAngleRatio
  Constant4 : Constant  Value=P_Global_CharSpd_ms
  Constant5 : Constant  Value=P_Global_WheelBase_m
  Constant6 : Constant  Value=57.3  OutDataTypeStr=single
  Enabled Subsystem : Subsystem  TreatAsAtomicUnit=on
  FilterTime2 : Product  Inputs=*//  RndMeth=Zero
  Logical Operator : Logic  AllPortsSameDT=off  OutDataTypeStr=boolean
  Memory52 : Memory  InheritSampleTime=on
  Sum : Sum  Inputs=+-
  Terminator : Terminator
  YOD_Ackman : MATLAB Function  TreatAsAtomicUnit=on
  SteerAngleOffset_deg : Outport
  wires:
  SteerAngle_deg/1 -> FilterTime2/1
  Compare To Constant1/1 -> Logical Operator/2
  YOD_Ackman/2(PsiDtAck) -> Memory52/1, Sum/1
  Enabled Subsystem/1(SteerAngleOffset_deg) -> SteerAngleOffset_deg/1  "LCS_LATC_CurrentSteerAngleOffset_deg"
  Constant5/1 -> YOD_Ackman/3(WheelBase)
  Constant4/1 -> YOD_Ackman/2(Vch)
  Memory52/1 -> YOD_Ackman/5(PsiDtAckK1)
  PsiDtOpt/1 -> Sum/2
  Bus Selector/1 -> YOD_Ackman/1(VxvRef), Compare To Constant1/1  "<LCS_Spd_ms>"
  Sum/1 -> Enabled Subsystem/2(Raw)
  Logical Operator/1 -> Enabled Subsystem/Enable, Terminator/1  "LCS_OffSetUpdate_Flg"
  Constant1/1 -> FilterTime2/2
  Constant6/1 -> FilterTime2/3
  YOD_Ackman/1(AckConst) -> Enabled Subsystem/1(AckConst)
  FilterTime2/1 -> YOD_Ackman/4(AlpWheelAngle)
  axvRef/1 -> Abs2/1
  Abs2/1 -> Compare To Constant6/1
  Compare To Constant6/1 -> Logical Operator/1
  Veh_Spd/1 -> Bus Selector/1

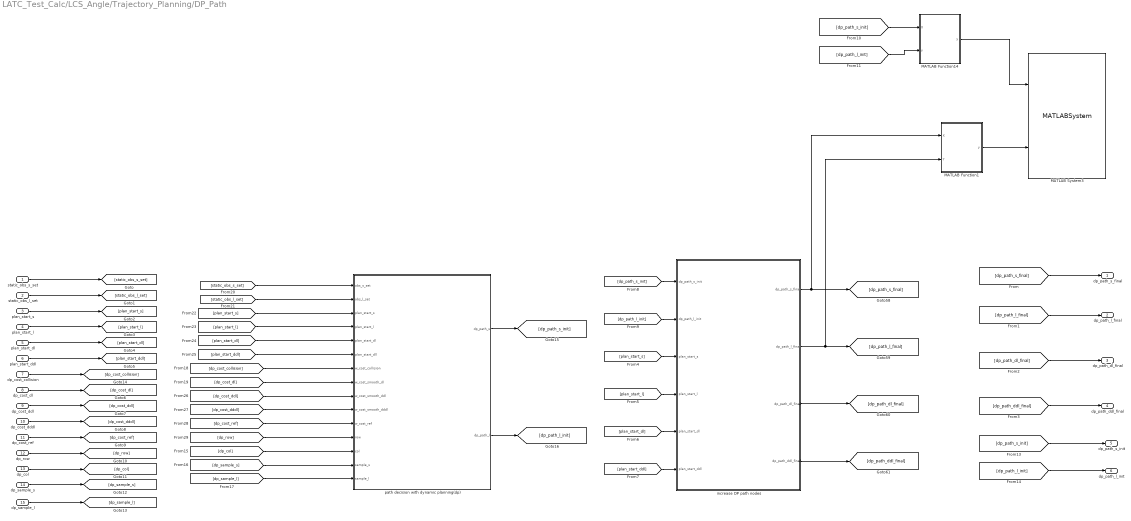
== system LATC_Test_Calc/LCS_Angle/Trajectory_Planning/DP_Path ==
  static_obs_s_set : Inport
  static_obs_l_set : Inport  Port=2
  plan_start_s : Inport  Port=3
  plan_start_l : Inport  Port=4
  plan_start_dl : Inport  Port=5
  plan_start_ddl : Inport  Port=6
  dp_cost_collision : Inport  Port=7
  dp_cost_dl : Inport  Port=8
  dp_cost_ddl : Inport  Port=9
  dp_cost_dddl : Inport  Port=10
  dp_cost_ref : Inport  Port=11
  dp_row : Inport  Port=12
  dp_col : Inport  Port=13
  dp_sample_s : Inport  Port=14
  dp_sample_l : Inport  Port=15
  MATLAB Function1 : MATLAB Function  TreatAsAtomicUnit=on
  MATLAB Function14 : MATLAB Function  TreatAsAtomicUnit=on
  MATLAB System3 : MATLABSystem  System=BirdsEyeView17a  XLim=[ 0, 120 ]  YLim=[ -30, 30 ]  HasActors=off  ActorsColor=off  HasVision=on  HasRadar=on  HasRoads=off  HasLaneMarkings=off  Camera_Fov=52  Camera_Range=100  Camera_Yaw=0  Camera_Pos=[ 0, 0 ]  Radar_Fov=52  Radar_Range=100  Radar_Yaw=0  Radar_Pos=[ 0, 0 ]  MarkerSize=4  LabelFontSize=4  LabelOffset=[ 1.5, 1.5 ]  aspectratio=off
      mask Type: BirdsEyeView17a
      mask Display:
      | disp(['Bird''s-Eye' char(10) 'View']);
      | port_label('input',1,'Vision');
      | port_label('input',2,'Radar');
  increase DP path nodes : MATLAB Function  TreatAsAtomicUnit=on
  path decision with dynamic planning(dp) : MATLAB Function  TreatAsAtomicUnit=on
  dp_path_s_final : Outport
  dp_path_l_final : Outport  Port=2
  dp_path_dl_final : Outport  Port=3
  dp_path_ddl_final : Outport  Port=4
  dp_path_s_init : Outport  Port=5
  dp_path_l_init : Outport  Port=6
  wires:
  [dp_path_s_final] -> dp_path_s_final/1
  [dp_path_l_final] -> dp_path_l_final/1
  [dp_path_dl_final] -> dp_path_dl_final/1
  [dp_path_ddl_final] -> dp_path_ddl_final/1
  dp_sample_l/1 -> [dp_sample_l]
  [dp_path_l_init] -> dp_path_l_init/1
  [dp_path_s_init] -> dp_path_s_init/1
  MATLAB Function14/1(y) -> MATLAB System3/1
  [static_obs_s_set] -> path decision with dynamic planning(dp)/1(obs_s_set)
  [static_obs_l_set] -> path decision with dynamic planning(dp)/2(obs_l_set)
  [plan_start_s] -> path decision with dynamic planning(dp)/3(plan_start_s)
  [plan_start_l] -> path decision with dynamic planning(dp)/4(plan_start_l)
  [plan_start_dl] -> path decision with dynamic planning(dp)/5(plan_start_dl)
  [plan_start_ddl] -> path decision with dynamic planning(dp)/6(plan_start_dll)
  [dp_cost_collision] -> path decision with dynamic planning(dp)/7(w_cost_collision)
  [dp_cost_dl] -> path decision with dynamic planning(dp)/8(w_cost_smooth_dl)
  [dp_cost_ddl] -> path decision with dynamic planning(dp)/9(w_cost_smooth_ddl)
  [dp_cost_dddl] -> path decision with dynamic planning(dp)/10(w_cost_smooth_dddl)
  [dp_cost_ref] -> path decision with dynamic planning(dp)/11(w_cost_ref)
  [dp_row] -> path decision with dynamic planning(dp)/12(row)
  [dp_col] -> path decision with dynamic planning(dp)/13(col)
  [dp_sample_s] -> path decision with dynamic planning(dp)/14(sample_s)
  [dp_sample_l] -> path decision with dynamic planning(dp)/15(sample_l)
  increase DP path nodes/1(dp_path_s_final) -> MATLAB Function1/1(X), [dp_path_s_final]
  increase DP path nodes/2(dp_path_l_final) -> MATLAB Function1/2(Y), [dp_path_l_final]
  MATLAB Function1/1(y) -> MATLAB System3/2
  increase DP path nodes/3(dp_path_dl_final) -> [dp_path_dl_final]
  increase DP path nodes/4(dp_path_ddl_final) -> [dp_path_ddl_final]
  [plan_start_s] -> increase DP path nodes/3(plan_start_s)
  [plan_start_l] -> increase DP path nodes/4(plan_start_l)
  [plan_start_dl] -> increase DP path nodes/5(plan_start_dl)
  [plan_start_ddl] -> increase DP path nodes/6(plan_start_ddl)
  static_obs_s_set/1 -> [static_obs_s_set]
  static_obs_l_set/1 -> [static_obs_l_set]
  plan_start_s/1 -> [plan_start_s]
  plan_start_l/1 -> [plan_start_l]
  plan_start_dl/1 -> [plan_start_dl]
  plan_start_ddl/1 -> [plan_start_ddl]
  dp_cost_collision/1 -> [dp_cost_collision]
  dp_cost_dl/1 -> [dp_cost_dl]
  dp_cost_ddl/1 -> [dp_cost_ddl]
  dp_cost_dddl/1 -> [dp_cost_dddl]
  dp_cost_ref/1 -> [dp_cost_ref]
  dp_row/1 -> [dp_row]
  dp_col/1 -> [dp_col]
  dp_sample_s/1 -> [dp_sample_s]
  path decision with dynamic planning(dp)/1(dp_path_s) -> [dp_path_s_init]
  path decision with dynamic planning(dp)/2(dp_path_l) -> [dp_path_l_init]
  [dp_path_s_init] -> increase DP path nodes/1(dp_path_s_init)
  [dp_path_l_init] -> increase DP path nodes/2(dp_path_l_init)
  [dp_path_s_init] -> MATLAB Function14/1(X)
  [dp_path_l_init] -> MATLAB Function14/2(Y)

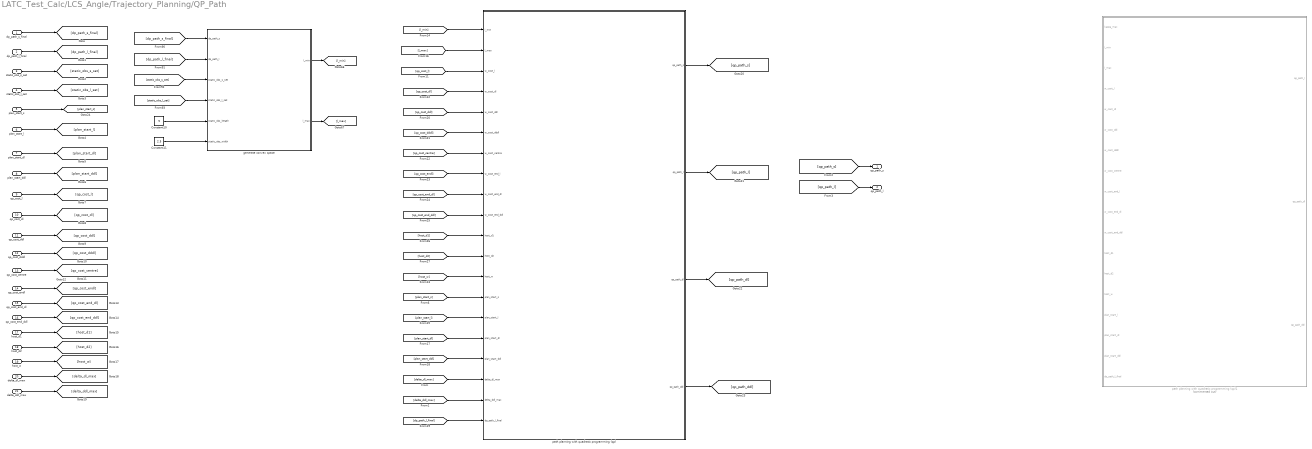
== system LATC_Test_Calc/LCS_Angle/Trajectory_Planning/QP_Path ==
  dp_path_s_final : Inport
  dp_path_l_final : Inport  Port=2
  static_obs_s_set : Inport  Port=3
  static_obs_l_set : Inport  Port=4
  plan_start_s : Inport  Port=5
  plan_start_l : Inport  Port=6
  plan_start_dl : Inport  Port=7
  plan_start_ddl : Inport  Port=8
  qp_cost_l : Inport  Port=9
  qp_cost_dl : Inport  Port=10
  qp_cost_ddl : Inport  Port=11
  qp_cost_dddl : Inport  Port=12
  qp_cost_centre : Inport  Port=13
  qp_cost_endl : Inport  Port=14
  qp_cost_end_dl : Inport  Port=15
  qp_cost_end_ddl : Inport  Port=16
  host_d1 : Inport  Port=17
  host_d2 : Inport  Port=18
  host_w : Inport  Port=19
  delta_dl_max : Inport  Port=20
  delta_ddl_max : Inport  Port=21
  Constant10 : Constant  Value=5  OutDataTypeStr=single
  Constant11 : Constant  Value=2.5  OutDataTypeStr=single
  generate convex space : MATLAB Function  TreatAsAtomicUnit=on
  path planning with quadratic programming (qp) : MATLAB Function  TreatAsAtomicUnit=on
  path planning with quadratic programming (qp)1 : MATLAB Function  Commented=on  TreatAsAtomicUnit=on
  qp_path_s : Outport
  qp_path_l : Outport  Port=2
  wires:
  generate convex space/2(l_max) -> [l_max]
  Constant11/1 -> generate convex space/6(static_obs_width)
  Constant10/1 -> generate convex space/5(static_obs_length)
  [static_obs_l_set] -> generate convex space/4(static_obs_l_set)
  [dp_path_s_final] -> generate convex space/1(dp_path_s)
  generate convex space/1(l_min) -> [l_min]
  [static_obs_s_set] -> generate convex space/3(static_obs_s_set)
  [dp_path_l_final] -> generate convex space/2(dp_path_l)
  dp_path_l_final/1 -> [dp_path_l_final]
  static_obs_s_set/1 -> [static_obs_s_set]
  static_obs_l_set/1 -> [static_obs_l_set]
  plan_start_l/1 -> [plan_start_l]
  plan_start_dl/1 -> [plan_start_dl]
  plan_start_ddl/1 -> [plan_start_ddl]
  qp_cost_l/1 -> [qp_cost_l]
  qp_cost_dl/1 -> [qp_cost_dl]
  qp_cost_ddl/1 -> [qp_cost_ddl]
  qp_cost_dddl/1 -> [qp_cost_dddl]
  qp_cost_centre/1 -> [qp_cost_centre]
  qp_cost_endl/1 -> [qp_cost_endl]
  qp_cost_end_dl/1 -> [qp_cost_end_dl]
  qp_cost_end_ddl/1 -> [qp_cost_end_ddl]
  host_d1/1 -> [host_d1]
  host_d2/1 -> [host_d2]
  host_w/1 -> [host_w]
  [host_w] -> path planning with quadratic programming (qp)/13(host_w)
  [host_d2] -> path planning with quadratic programming (qp)/12(host_d2)
  [host_d1] -> path planning with quadratic programming (qp)/11(host_d1)
  [qp_cost_end_ddl] -> path planning with quadratic programming (qp)/10(w_cost_end_ddl)
  [qp_cost_end_dl] -> path planning with quadratic programming (qp)/9(w_cost_end_dl)
  [qp_cost_endl] -> path planning with quadratic programming (qp)/8(w_cost_end_l)
  [qp_cost_centre] -> path planning with quadratic programming (qp)/7(w_cost_centre)
  [qp_cost_dddl] -> path planning with quadratic programming (qp)/6(w_cost_dddl)
  [qp_cost_ddl] -> path planning with quadratic programming (qp)/5(w_cost_ddl)
  [qp_cost_dl] -> path planning with quadratic programming (qp)/4(w_cost_dl)
  [qp_cost_l] -> path planning with quadratic programming (qp)/3(w_cost_l)
  [plan_start_l] -> path planning with quadratic programming (qp)/15(plan_start_l)
  [plan_start_dl] -> path planning with quadratic programming (qp)/16(plan_start_dl)
  [plan_start_ddl] -> path planning with quadratic programming (qp)/17(plan_start_ddl)
  [l_min] -> path planning with quadratic programming (qp)/1(l_min)
  [l_max] -> path planning with quadratic programming (qp)/2(l_max)
  dp_path_s_final/1 -> [dp_path_s_final]
  delta_dl_max/1 -> [delta_dl_max]
  delta_ddl_max/1 -> [delta_ddl_max]
  [delta_dl_max] -> path planning with quadratic programming (qp)/18(delta_dl_max)
  [delta_ddl_max] -> path planning with quadratic programming (qp)/19(delta_ddl_max)
  path planning with quadratic programming (qp)/1(qp_path_s) -> [qp_path_s]
  path planning with quadratic programming (qp)/2(qp_path_l) -> [qp_path_l]
  path planning with quadratic programming (qp)/3(qp_path_dl) -> [qp_path_dl]
  path planning with quadratic programming (qp)/4(qp_path_ddl) -> [qp_path_ddl]
  [qp_path_s] -> qp_path_s/1
  [qp_path_l] -> qp_path_l/1
  [plan_start_s] -> path planning with quadratic programming (qp)/14(plan_start_s)
  plan_start_s/1 -> [plan_start_s]
  [dp_path_l_final] -> path planning with quadratic programming (qp)/20(dp_path_l_final)

== system LATC_Test_Calc/LCS_Angle/Trajectory_Points/RoadCreate1 ==
  A0 : Inport  OutDataTypeStr=single
  A1 : Inport  Port=2
  A2 : Inport  Port=3
  A3 : Inport  Port=4
  LineVaild : Inport  Port=5
  Constant25 : Constant  Value=P_LCS_LineVaildSW
  Constant33 : Constant  Value=0  OutDataTypeStr=boolean
  MATLAB Function1 : MATLAB Function  TreatAsAtomicUnit=on
  Switch2 : Switch  Criteria=u2 > Threshold
  CenterLinePointX : Outport
  CenterLinePointY : Outport  Port=2
  Control_Valid : Outport  Port=3  OutDataTypeStr=boolean
  wires:
  A0/1 -> MATLAB Function1/1(A0)
  A1/1 -> MATLAB Function1/2(A1)
  A3/1 -> MATLAB Function1/4(A3)
  A2/1 -> MATLAB Function1/3(A2)
  Switch2/1 -> Control_Valid/1
  Constant33/1 -> Switch2/1
  LineVaild/1 -> Switch2/3
  Constant25/1 -> Switch2/2
  MATLAB Function1/1(CenterLinePointX) -> CenterLinePointX/1
  MATLAB Function1/2(CenterLinePointY) -> CenterLinePointY/1

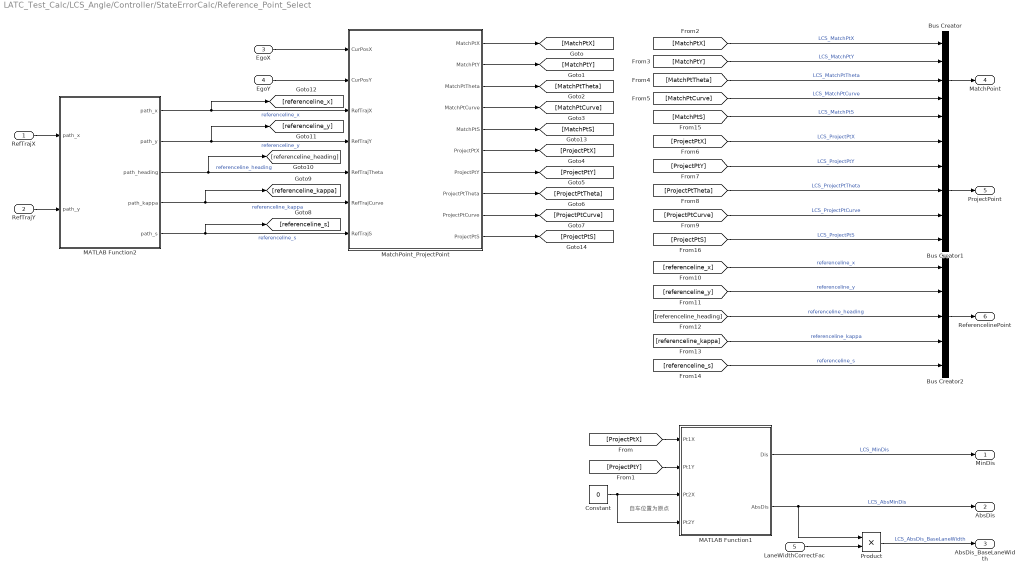
== system LATC_Test_Calc/LCS_Angle/Controller/StateErrorCalc/Reference_Point_Select ==
  note: 自车位置为原点
  RefTrajX : Inport
  RefTrajY : Inport  Port=2
  EgoX : Inport  Port=3
  EgoY : Inport  Port=4
  LaneWidthCorrectFac : Inport  Port=5
  Bus Creator : BusCreator  Inputs=5
  Bus Creator1 : BusCreator  Inputs=5
  Bus Creator2 : BusCreator  Inputs=5
  Constant : Constant  Value=0  OutDataTypeStr=single
  MATLAB Function1 : MATLAB Function  TreatAsAtomicUnit=on
  MATLAB Function2 : MATLAB Function  TreatAsAtomicUnit=on
  MatchPoint_ProjectPoint : MATLAB Function  TreatAsAtomicUnit=on
  Product : Product
  MinDis : Outport
  AbsDis : Outport  Port=2
  AbsDis_BaseLaneWidth : Outport  Port=3
  MatchPoint : Outport  Port=4
  ProjectPoint : Outport  Port=5
  ReferencelinePoint : Outport  Port=6
  wires:
  EgoX/1 -> MatchPoint_ProjectPoint/1(CurPosX)
  EgoY/1 -> MatchPoint_ProjectPoint/2(CurPosY)
  MATLAB Function1/1(Dis) -> MinDis/1  "LCS_MinDis"
  MATLAB Function1/2(AbsDis) -> AbsDis/1, Product/1  "LCS_AbsMinDis"
  LaneWidthCorrectFac/1 -> Product/2
  Product/1 -> AbsDis_BaseLaneWidth/1  "LCS_AbsDis_BaseLaneWidth"
  MATLAB Function2/1(path_x) -> MatchPoint_ProjectPoint/3(RefTrajX), [referenceline_x]  "referenceline_x"
  MATLAB Function2/2(path_y) -> MatchPoint_ProjectPoint/4(RefTrajY), [referenceline_y]  "referenceline_y"
  MATLAB Function2/3(path_heading) -> MatchPoint_ProjectPoint/5(RefTrajTheta), [referenceline_heading]  "referenceline_heading"
  MATLAB Function2/4(path_kappa) -> MatchPoint_ProjectPoint/6(RefTrajCurve), [referenceline_kappa]  "referenceline_kappa"
  MATLAB Function2/5(path_s) -> MatchPoint_ProjectPoint/7(RefTrajS), [referenceline_s]  "referenceline_s"
  RefTrajY/1 -> MATLAB Function2/2("path_y ")
  RefTrajX/1 -> MATLAB Function2/1("path_x ")
  MatchPoint_ProjectPoint/1(MatchPtX) -> [MatchPtX]
  MatchPoint_ProjectPoint/2(MatchPtY) -> [MatchPtY]
  MatchPoint_ProjectPoint/3(MatchPtTheta) -> [MatchPtTheta]
  MatchPoint_ProjectPoint/4(MatchPtCurve) -> [MatchPtCurve]
  MatchPoint_ProjectPoint/6(ProjectPtX) -> [ProjectPtX]
  MatchPoint_ProjectPoint/7(ProjectPtY) -> [ProjectPtY]
  MatchPoint_ProjectPoint/8(ProjectPtTheta) -> [ProjectPtTheta]
  MatchPoint_ProjectPoint/9(ProjectPtCurve) -> [ProjectPtCurve]
  Constant/1 -> MATLAB Function1/4(Pt2Y), MATLAB Function1/3(Pt2X)
  [ProjectPtX] -> MATLAB Function1/1(Pt1X)
  [ProjectPtY] -> MATLAB Function1/2(Pt1Y)
  [MatchPtX] -> Bus Creator/1  "LCS_MatchPtX"
  [MatchPtY] -> Bus Creator/2  "LCS_MatchPtY"
  [MatchPtTheta] -> Bus Creator/3  "LCS_MatchPtTheta"
  [MatchPtCurve] -> Bus Creator/4  "LCS_MatchPtCurve"
  Bus Creator/1 -> MatchPoint/1
  Bus Creator1/1 -> ProjectPoint/1
  [ProjectPtCurve] -> Bus Creator1/4  "LCS_ProjectPtCurve"
  [ProjectPtTheta] -> Bus Creator1/3  "LCS_ProjectPtTheta"
  [ProjectPtY] -> Bus Creator1/2  "LCS_ProjectPtY"
  [ProjectPtX] -> Bus Creator1/1  "LCS_ProjectPtX"
  [referenceline_x] -> Bus Creator2/1  "referenceline_x"
  [referenceline_y] -> Bus Creator2/2  "referenceline_y"
  [referenceline_heading] -> Bus Creator2/3  "referenceline_heading"
  [referenceline_kappa] -> Bus Creator2/4  "referenceline_kappa"
  Bus Creator2/1 -> ReferencelinePoint/1
  [referenceline_s] -> Bus Creator2/5  "referenceline_s"
  MatchPoint_ProjectPoint/5(MatchPtS) -> [MatchPtS]
  MatchPoint_ProjectPoint/10(ProjectPtS) -> [ProjectPtS]
  [MatchPtS] -> Bus Creator/5  "LCS_MatchPtS"
  [ProjectPtS] -> Bus Creator1/5  "LCS_ProjectPtS"

== system LATC_Test_Calc/LCS_Angle/Controller/TargetAngleCalc/Median_Filter ==
  In : Inport
  Constant11 : Constant  Value=P_LCS_LATC_TarAngleFliterWindowSize - single(2)  OutDataTypeStr=single
  Divide1 : Product  Inputs=*/
  Max of Elements1 : MinMax  Function=max
  MinMax2 : MinMax
  Minus1 : Sum  Inputs=--+
  Sum of Elements1 : Sum  Inputs=+
  Tapped Delay1 : simulink/Discrete/Tapped Delay  vinit=0.0  samptime=-1  NumDelays=P_LCS_LATC_TarAngleFliterWindowSize-1  DelayOrder=Newest  includeCurrent=on
  Out : Outport
  wires:
  Max of Elements1/1 -> Minus1/2
  Divide1/1 -> Out/1
  Minus1/1 -> Divide1/1
  In/1 -> Tapped Delay1/1
  MinMax2/1 -> Minus1/1
  Sum of Elements1/1 -> Minus1/3
  Tapped Delay1/1 -> Max of Elements1/1, MinMax2/1, Sum of Elements1/1
  Constant11/1 -> Divide1/2
